simulink model "controle"  (R2018a)
settings: Solver=VariableStepAuto  StartTime=0.0  StopTime=30  RelTol=1e-3
values from neighbouring files (symbols this model uses):
  k1 = 6.01    [setup6.m]
  k2 = 0.8433    [setup6.m]
  k3 = 0.1123    [setup6.m]
settings Model: Creator=crist  LastModifiedBy=crist

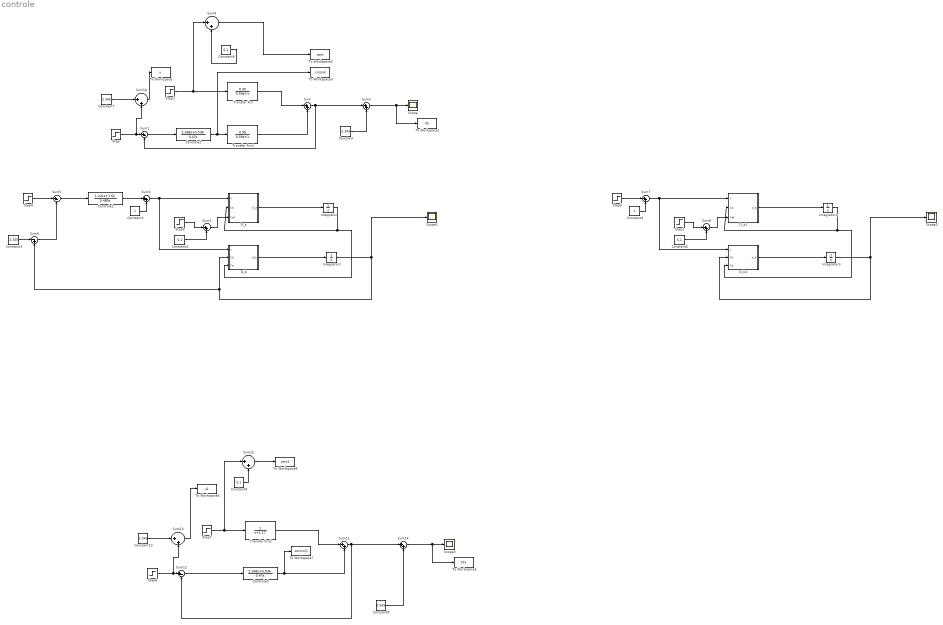
== system controle ==
  Constant{,3,7..8,10} (5 alike) : Constant  Value=2.345
  Constant1 : Constant
  Constant{2,5..6,9} (4 alike) : Constant  Value=5.1
  Constant4 : Constant
  Controle1 : TransferFcn  Numerator=[1.241 1.62]  Denominator=[0.485 0]
  Controle2 : TransferFcn  Numerator=[2.168 4.536]  Denominator=[0.47 0]
  Controle3 : TransferFcn  Numerator=[2.168 4.536]  Denominator=[0.47 0]
  D_a : MATLAB Function  TreatAsAtomicUnit=on
  D_a1 : MATLAB Function  TreatAsAtomicUnit=on
  D_b : MATLAB Function  TreatAsAtomicUnit=on
  D_b1 : MATLAB Function  TreatAsAtomicUnit=on
  Integrator : Integrator  InitialCondition=0.7192
  Integrator1 : Integrator  InitialCondition=2.345
  Integrator2 : Integrator
  Integrator3 : Integrator
  Scope{,1..3} (4 alike) : Scope
  Step : Step  Time=10  After=0.2  SampleTime=0
  Step1 : Step  Time=20  After=0.3  SampleTime=0
  Step2 : Step  Time=10  After=0.3  SampleTime=0
  Step3 : Step  Time=35  After=0.2  SampleTime=0
  Step4 : Step  Time=20  After=0.3  SampleTime=0
  Step5 : Step  Time=10  After=0  SampleTime=0
  Step6 : Step  Time=10  After=0.2  SampleTime=0
  Step7 : Step  Time=20  After=0.3  SampleTime=0
  Sum{,2..4,7..11,13..15} (12 alike) : Sum  Inputs=|++
  Sum1 : Sum  Inputs=|+-
  Sum12 : Sum  Inputs=|+-
  Sum5 : Sum  Inputs=|+-
  Sum6 : Sum  Inputs=|-+
  To Workspace : ToWorkspace  VariableName=u  SaveFormat=Timeseries  SampleTime=-1
  To Workspace1 : ToWorkspace  VariableName=Cb  SaveFormat=Timeseries  SampleTime=-1
  To Workspace2 : ToWorkspace  VariableName=pert  SaveFormat=Timeseries  SampleTime=-1
  To Workspace3 : ToWorkspace  VariableName=control  SaveFormat=Timeseries  SampleTime=-1
  To Workspace4 : ToWorkspace  VariableName=u1  SaveFormat=Timeseries  SampleTime=-1
  To Workspace5 : ToWorkspace  VariableName=Cb1  SaveFormat=Timeseries  SampleTime=-1
  To Workspace6 : ToWorkspace  VariableName=pert1  SaveFormat=Timeseries  SampleTime=-1
  To Workspace7 : ToWorkspace  VariableName=control1  SaveFormat=Timeseries  SampleTime=-1
  Transfer Fcn : TransferFcn  Numerator=[0.45]  Denominator=[0.59 1]
  Transfer Fcn1 : TransferFcn  Numerator=[0.56]  Denominator=[0.59 1]
  Transfer Fcn2 : TransferFcn  Denominator=[1 1.17]
  wires:
  Transfer Fcn1/1 -> Sum/2
  Transfer Fcn/1 -> Sum/1
  Controle2/1 -> To Workspace3/1, Transfer Fcn1/1
  Sum1/1 -> Controle2/1
  Sum/1 -> Sum2/1, Sum1/2
  Step/1 -> Sum10/2, Sum1/1
  Step1/1 -> Sum9/1, Transfer Fcn/1
  Constant/1 -> Sum2/2
  Sum2/1 -> To Workspace1/1, Scope/1
  Constant2/1 -> Sum4/2
  Sum3/1 -> D_b/1(u), D_a/1(u)
  Sum4/1 -> D_a/3(Caf)
  Integrator/1 -> D_b/3(Ca), D_a/2(Ca)
  Constant1/1 -> Sum3/2
  D_a/1(d_a) -> Integrator/1
  Integrator1/1 -> Scope1/1, Sum6/2, D_b/2(Cb)
  Step3/1 -> Sum4/1
  D_b/1(d_b) -> Integrator1/1
  Sum5/1 -> Controle1/1
  Step4/1 -> Sum5/1
  Controle1/1 -> Sum3/1
  Constant3/1 -> Sum6/1
  Sum6/1 -> Sum5/2
  Sum7/1 -> D_b1/1(u), D_a1/1(u)
  Step2/1 -> Sum8/1
  D_b1/1(d_b) -> Integrator3/1
  Constant4/1 -> Sum7/2
  Integrator2/1 -> D_b1/3(Ca), D_a1/2(Ca)
  Step5/1 -> Sum7/1
  D_a1/1(d_a) -> Integrator2/1
  Sum8/1 -> D_a1/3(Caf)
  Integrator3/1 -> Scope2/1, D_b1/2(Cb)
  Constant5/1 -> Sum8/2
  Constant6/1 -> Sum9/2
  Sum9/1 -> To Workspace2/1
  Sum10/1 -> To Workspace/1
  Constant7/1 -> Sum10/1
  Sum13/1 -> To Workspace4/1
  Constant10/1 -> Sum13/1
  Constant8/1 -> Sum14/2
  Sum15/1 -> To Workspace6/1
  Constant9/1 -> Sum15/2
  Controle3/1 -> Sum11/2, To Workspace7/1
  Sum14/1 -> To Workspace5/1, Scope3/1
  Step7/1 -> Transfer Fcn2/1, Sum15/1
  Sum11/1 -> Sum14/1, Sum12/2
  Transfer Fcn2/1 -> Sum11/1
  Step6/1 -> Sum13/2, Sum12/1
  Sum12/1 -> Controle3/1

== matlab function controle/D_a ==
  data: u input; d_a output; Ca input; Caf input; k1 parameter; k3 parameter
function d_a = fcn(u,Ca,Caf, k1, k3)

d_a = -k1*Ca - k3*Ca^2 + (Caf-Ca)*u;

== matlab function controle/D_b ==
  data: u input; d_b output; Cb input; Ca input; k1 parameter; k2 parameter
function d_b = fcn(u,Cb,Ca, k1, k2)

d_b = k1*Ca - k2*Cb - Cb*u;

== matlab function controle/D_a1 ==
  data: u input; d_a output; Ca input; Caf input; k1 parameter; k3 parameter
function d_a = fcn(u,Ca,Caf, k1, k3)

d_a = -k1*Ca - k3*Ca^2 + (Caf-Ca)*u;

== matlab function controle/D_b1 ==
  data: u input; d_b output; Cb input; Ca input; k1 parameter; k2 parameter
function d_b = fcn(u,Cb,Ca, k1, k2)

d_b = k1*Ca - k2*Cb - Cb*u;
